simulink model "Lab7_DCMotorControl"  (R2017a)
settings: Solver=VariableStepAuto  StartTime=0.0  StopTime=10  RelTol=1e-3
settings Model: Creator=jfrancis  LastModifiedBy=jfrancis

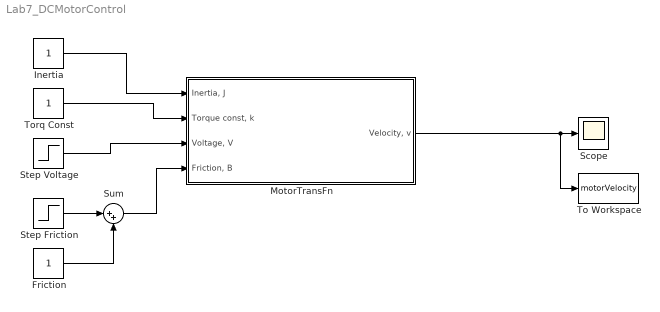
== system Lab7_DCMotorControl ==
  Friction : Constant
  Inertia : Constant
  MotorTransFn : Subsystem
  Scope : Scope
  Step Friction : Step  Time=5  SampleTime=0
  Step Voltage : Step  SampleTime=0
  Sum : Sum  Inputs=|++
  To Workspace : ToWorkspace  VariableName=motorVelocity  SaveFormat=Timeseries  SampleTime=-1
  Torq Const : Constant
  wires:
  Inertia/1 -> MotorTransFn/1("Inertia, J")
  Torq Const/1 -> MotorTransFn/2("Torque const, k")
  Step Friction/1 -> Sum/1
  Friction/1 -> Sum/2
  Sum/1 -> MotorTransFn/4("Friction, B")
  Step Voltage/1 -> MotorTransFn/3("Voltage, V")
  MotorTransFn/1("Velocity, v") -> To Workspace/1, Scope/1

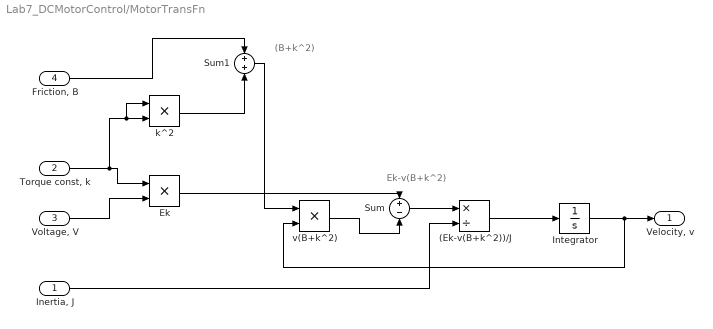
== system Lab7_DCMotorControl/MotorTransFn ==
  note: Ek-v(B+k^2)
  note: (B+k^2)
  "Inertia, J" : Inport
  "Torque const, k" : Inport  Port=2
  "Voltage, V" : Inport  Port=3
  "Friction, B" : Inport  Port=4
  (Ek-v(B+k^2))/J : Product  Inputs=*/
  Ek : Product
  Integrator : Integrator
  Sum : Sum  Inputs=+-
  Sum1 : Sum
  k^2 : Product
  v(B+k^2) : Product
  "Velocity, v" : Outport
  wires:
  Ek/1 -> Sum/1
  "Friction, B"/1 -> Sum1/1
  (Ek-v(B+k^2))/J/1 -> Integrator/1
  Sum1/1 -> v(B+k^2)/1
  "Voltage, V"/1 -> Ek/2
  "Inertia, J"/1 -> (Ek-v(B+k^2))/J/2
  k^2/1 -> Sum1/2
  Sum/1 -> (Ek-v(B+k^2))/J/1
  "Torque const, k"/1 -> k^2/1, k^2/2, Ek/1
  Integrator/1 -> v(B+k^2)/2, "Velocity, v"/1
  v(B+k^2)/1 -> Sum/2
